simulink model "Resilient-MPC"  (R2018b)
settings: Solver=VariableStepAuto  StartTime=0.0  StopTime=10  RelTol=1e-3
values from neighbouring files (symbols this model uses):
  F = [F,S]    [Initialization.m]
  O = [O;(C*A^(i-1))]    [Initialization.m]
  p = kron(L,pp)    [Initialization.m]
undefined symbols (not defined in the file or in its folder): sigbuilder_block
settings Model: Creator=lenovo  LastModifiedBy=lenovo

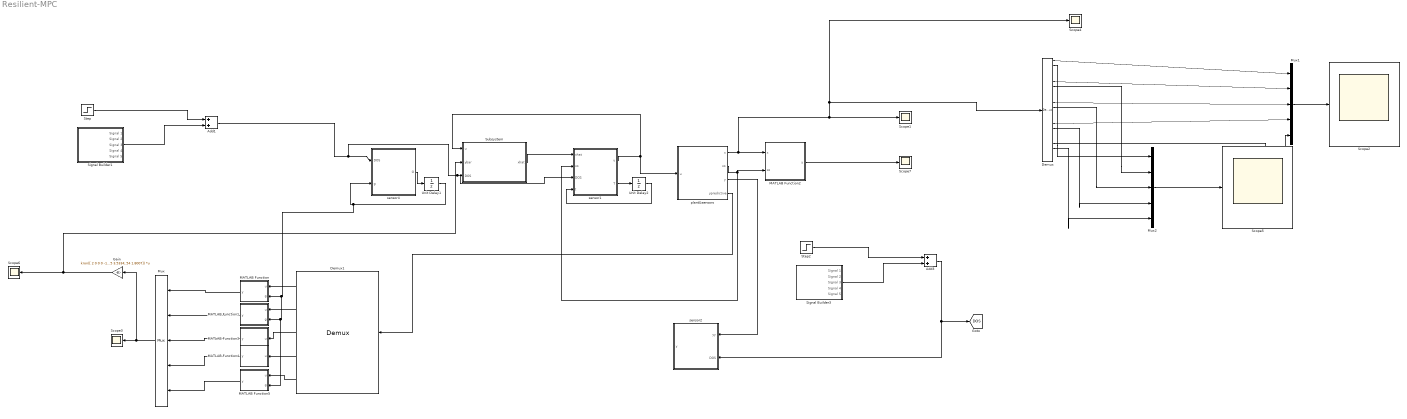
== system Resilient-MPC ==
  Add1 : Sum
  Add3 : Sum
  Demux : Demux  Outputs=20
  Demux1 : Demux  Outputs=5
  Gain : Gain  Gain=kron([ 2 0 0 0 -1; -1 2 0 0 0; -1 0 1 0 0; 0 -1 0 1 0; 0 -1 -1 -1 3],[3.0849 0.6931;2.4258 34.9384;7.0235 3.5334;.54 1.8007])  Multiplication=Matrix(K*u)
  MATLAB Function : MATLAB Function  TreatAsAtomicUnit=on
  MATLAB Function1 : MATLAB Function  TreatAsAtomicUnit=on
  MATLAB Function2 : MATLAB Function  TreatAsAtomicUnit=on
  MATLAB Function3 : MATLAB Function  TreatAsAtomicUnit=on
  MATLAB Function4 : MATLAB Function  TreatAsAtomicUnit=on
  MATLAB Function5 : MATLAB Function  TreatAsAtomicUnit=on
  Mux : Mux  Inputs=5
  Mux1 : Mux  Inputs=5
  Mux2 : Mux  Inputs=5
  Scope{1..7} (7 alike) : Scope
  Signal Builder1 : Subsystem  Tag=STV Subsys  LoadFcn=sigbuilder_block('load');  StartFcn=sigbuilder_block('start');  StopFcn=sigbuilder_block('stop');  ClipboardFcn=sigbuilder_block('clipboard');  mask(Sigbuilder block){tuvar=[0:10]}
      mask help: Simulink:masks:SigbuilderBlock_MD
      mask init:
      | if ~strcmp(get_param(bdroot(gcbh),'SimulationStatus'),'stopped') tuvar = sigbuilder_block('maskInit'); end
      settings: CopyFcn=sigbuilder_block('copy');  DeleteFcn=sigbuilder_block('delete');  ModelCloseFcn=sigbuilder_block('modelClose');  PreSaveFcn=sigbuilder_block('preSave');  PauseFcn=sigbuilder_block('pause');  ContinueFcn=sigbuilder_block('continue');  NameChangeFcn=sigbuilder_block('namechange');  OpenFcn=sigbuilder_block('open',[5.4 30 1141.2 522.6 ]);  CloseFcn=sigbuilder_block('close');
      mask Display: plot(0, 0, 100, 100,[2, 2, 32, 32, 2], [68, 8, 8, 68, 68],[32, 2], [38, 38], [32, 19, 2],[53, 60, 44], [32, 17, 17, 2],[16, 16, 31, 31]);txt = getActiveGroup(gcbh);text(2, 100, txt,'verticalAlignment', 'top');
  Signal Builder3 : Subsystem  Tag=STV Subsys  LoadFcn=sigbuilder_block('load');  StartFcn=sigbuilder_block('start');  StopFcn=sigbuilder_block('stop');  ClipboardFcn=sigbuilder_block('clipboard');  mask(Sigbuilder block){tuvar=[0:10]}
      mask help: Simulink:masks:SigbuilderBlock_MD
      mask init:
      | if ~strcmp(get_param(bdroot(gcbh),'SimulationStatus'),'stopped') tuvar = sigbuilder_block('maskInit'); end
      settings: CopyFcn=sigbuilder_block('copy');  DeleteFcn=sigbuilder_block('delete');  ModelCloseFcn=sigbuilder_block('modelClose');  PreSaveFcn=sigbuilder_block('preSave');  PauseFcn=sigbuilder_block('pause');  ContinueFcn=sigbuilder_block('continue');  NameChangeFcn=sigbuilder_block('namechange');  OpenFcn=sigbuilder_block('open',[5.4 30 1141.2 522.6 ]);  CloseFcn=sigbuilder_block('close');
      mask Display: plot(0, 0, 100, 100,[2, 2, 32, 32, 2], [68, 8, 8, 68, 68],[32, 2], [38, 38], [32, 19, 2],[53, 60, 44], [32, 17, 17, 2],[16, 16, 31, 31]);txt = getActiveGroup(gcbh);text(2, 100, txt,'verticalAlignment', 'top');
  Step : Step  After=-1  SampleTime=10
  Step2 : Step  After=-1  SampleTime=10
  Subsystem : Subsystem
  Unit Delay1 : UnitDelay  InitialCondition=[eye(2) zeros(2,6)]  SampleTime=0.01
  Unit Delay2 : UnitDelay  InitialCondition=[1 0 0 0]  SampleTime=0.01
  plant&sensors : Subsystem
  sensor1 : MATLAB Function  TreatAsAtomicUnit=on
  sensor2 : MATLAB Function  TreatAsAtomicUnit=on
  sensor4 : MATLAB Function  TreatAsAtomicUnit=on
  tag scope: DOS=global
  wires:
  MATLAB Function2/1(y) -> Scope7/1
  sensor1/1(u) -> plant&sensors/1(u), Subsystem/1(u)
  Subsystem/1(xhat) -> sensor1/1(xhat)
  plant&sensors/3(y) -> sensor2/1(yy)
  plant&sensors/2(xo) -> MATLAB Function2/2(xo), sensor1/2(xo)
  Add1/1 -> sensor1/3(DOS), Subsystem/3(DOS), sensor4/1(DOS)
  plant&sensors/4(ypredictive) -> Demux1/1
  sensor4/1(G) -> Unit Delay1/1
  Unit Delay1/1 -> MATLAB Function5/2(g), MATLAB Function1/2(g), MATLAB Function/2(g), sensor4/2(g)
  plant&sensors/1(x) -> Demux/1, Scope4/1, Scope1/1, MATLAB Function2/1(x)
  sensor1/2(T) -> Unit Delay2/1
  Unit Delay2/1 -> sensor1/4(t)
  Step2/1 -> Add3/1
  Signal Builder3/3(Signal 3) -> Add3/2
  Add3/1 -> [DOS], sensor2/2(DOS)
  Step/1 -> Add1/1
  Signal Builder1/3(Signal 3) -> Add1/2
  Demux1/1 -> MATLAB Function/1(u)
  Demux1/2 -> MATLAB Function1/1(u)
  Demux1/3 -> MATLAB Function3/1(u)
  Demux1/4 -> MATLAB Function4/1(u)
  Demux1/5 -> MATLAB Function5/1(u)
  MATLAB Function/1(y) -> Mux/1
  MATLAB Function1/1(y) -> Mux/2
  MATLAB Function3/1(y) -> Mux/3
  MATLAB Function4/1(y) -> Mux/4
  MATLAB Function5/1(y) -> Mux/5
  Mux/1 -> Gain/1, Scope3/1
  Gain/1 -> Subsystem/2(ybar), Scope6/1
  Demux/5 -> Mux1/2
  Demux/17 -> Mux1/5
  Mux1/1 -> Scope2/1
  Demux/13 -> Mux1/4
  Demux/1 -> Mux1/1
  Demux/14 -> Mux2/4
  Demux/9 -> Mux1/3
  Demux/6 -> Mux2/2
  Demux/2 -> Mux2/1
  Demux/10 -> Mux2/3
  Mux2/1 -> Scope5/1
  Demux/18 -> Mux2/5

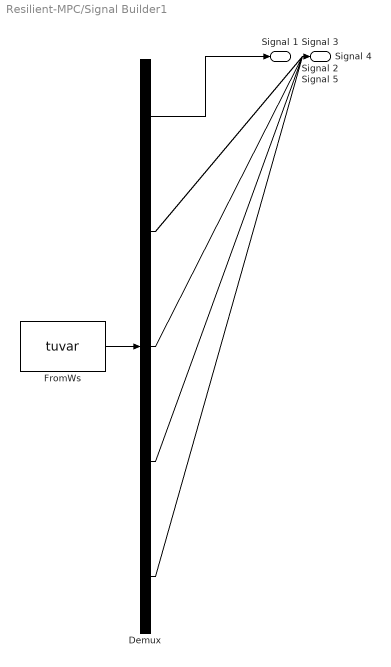
== system Resilient-MPC/Signal Builder1 ==
  Demux : Demux  Tag=STV Demux  Outputs=5
  FromWs : FromWorkspace  Tag=STV FromWs  VariableName=tuvar  SampleTime=0
      SigBuilderData=|
      | common.afterFinalStr = 'Extrapolate'
      | common.sampleTime = 0
      | dataSet.timeRange = [0 10]
      | dataSet.name = 'Group 1'
      | sbobj.Groups.Name = 'Group 1'
      | sbobj.Groups.Signals(1).Name = 'Signal 1'
      | sbobj.Groups.Signals(1).XData = [0 4 4 6 6 10]
      | sbobj.Groups.Signals(1).YData = [0 0 1 1 0 0]
      | sbobj.Groups.Signals(2).Name = 'Signal 2'
      | sbobj.Groups.Signals(2).XData = [0 0.125 0.125 0.25 0.25 0.375 0.375 0.5 0.5 0.625 0.625 0.75 0.75 0.875 0.875 1 1 1.125 1.125 1.25 1.25 1.375 1.375 1.5 1.5 1.625 1.625 1.75 1.75 1.875 1.875 2 2 2.125 2.125 2.25 2.25 2.375 2.375 2.5 2.5 2.625 2.625 2.75 2.75 2.875 2.875 3 3 3.125 3.125 3.25 3.25 3.375 3.375 3.5 3.5 3.625 3.625 3.75 3.75 3.875 3.875 4 4 4.125 4.125 4.25 4.25 4.375 4.375 4.5 4.5 4.625 4.625 4.75 4.75 4.875 4.875 5 5 5.125 5.125 5.25 5.25 5.375 5.375 5.5 5.5 5.625 5.625 5.75 5.75 5.875 5.875 6 6 6.125 6.125 6.25 6.25 6.375 6.375 6.5 6.5 6.625 6.625 6.75 6.75 6.875 6.875 7 7 7.125 7.125 7.25 7.25 7.375 7.375 7.5 7.5 7.625 7.625 7.75 7.75 7.875 7.875 8 8 8.125 8.125 8.25 8.25 8.375 8.375 8.5 8.5 8.625 8.625 8.75 8.75 8.875 8.875 9 9 9.125 9.125 9.25 9.25 9.375 9.375 9.5 9.5 9.625 9.625 9.75 9.75 9.875 9.875 10]
      | sbobj.Groups.Signals(2).YData = [1 1 -1 -1 1 1 -1 -1 1 1 -1 -1 1 1 -1 -1 1 1 -1 -1 1 1 -1 -1 1 1 -1 -1 1 1 -1 -1 1 1 -1 -1 1 1 -1 -1 1 1 -1 -1 1 1 -1 -1 1 1 -1 -1 1 1 -1 -1 1 1 -1 -1 1 1 -1 -1 1 1 -1 -1 1 1 -1 -1 1 1 -1 -1 1 1 -1 -1 1 1 -1 -1 1 1 -1 -1 1 1 -1 -1 1 1 -1 -1 1 1 -1 -1 1 1 -1 -1 1 1 -1 -1 1 1 -1 -1 1 1 -1 -1 1 1 -1 -1 1 1 -1 -1 1 1 -1 -1 1 1 -1 -1 1 1 -1 -1 1 1 -1 -1 1 1 -1 -1 1 1 -1 -1 1 1 -1 -1 1 1 -1 -1 1 1 -1 -1]
      | sbobj.Groups.Signals(3).Name = 'Signal 3'
      | sbobj.Groups.Signals(3).XData = [0 0.16 0.333333333333 0.4 0.4 0.46 0.46 0.833333333333 1 1.005 1.005 1.3 1.3 1.8 1.8 1.9 1.9 2.4 2.4 2.55 2.55 2.625 2.785 2.83333333333 3 3.2 3.2 3.4 3.4 3.5 3.66666666667 3.83333333333 4 4 4.17 4.17 4.33333333333 4.5 4.8 4.8 4.85 4.85 5 5.16666666667 5.33333333333 5.33333333333 5.5 5.5 5.66666666667 5.83333333333 5.83333333333 6 6 6.16666666667 6.33333333333 6.5 6.5 6.66666666667 6.66666666667 6.83333333333 7 7 7.16666666667 7.16666666667 7.33333333333 7.5 7.66666666667 7.83333333333 7.83333333333 8 8 8.16666666667 8.33333333333 8.5 8.5 8.66666666667 8.66666666667 8.83333333333 9 9.16666666667 9.33333333333 9.33333333333 9.5 9.5 9.66666666667 9.83333333333 10]
      | sbobj.Groups.Signals(3).YData = [1 1 1 1 0 0 1 1 1 1 0 0 1 1 0 0 1 1 0 0 1 1 1 1 1 1 0 0 1 1 1 1 1 0 0 1 1 1 1 0 0 1 1 1 1 0 0 1 1 1 0 0 1 1 1 1 0 0 1 1 1 0.005 0.005 1 1 1 1 1 0 0 1 1 1 1 0 0 1 1 1 1 1 0 0 1 1 1 1]
      | sbobj.Groups.Signals(4).Name = 'Signal 4'
      | sbobj.Groups.Signals(4).XData = [0 5 5 10]
      | sbobj.Groups.Signals(4).YData = [0 0 1 1]
      | sbobj.Groups.Signals(5).Name = 'Signal 5'
      | sbobj.Groups.Signals(5).XData = [0 0.45 0.45 0.5 0.5 0.95 0.95 1 1 1.45 1.45 1.5 1.5 1.95 1.95 2 2 2.45 2.45 2.5 2.5 2.95 2.95 3 3 3.45 3.45 3.5 3.5 3.95 3.95 4 4 4.45 4.45 4.5 4.5 4.95 4.95 5 5 5.45 5.45 5.5 5.5 5.95 5.95 6 6 6.45 6.45 6.5 6.5 6.95 6.95 7 7 7.45 7.45 7.5 7.5 7.95 7.95 8 8 8.45 8.45 8.5 8.5 8.95 8.95 9 9 9.45 9.45 9.5 9.5 9.95 9.95 10]
      | sbobj.Groups.Signals(5).YData = [1 1 0 0 1 1 0 0 1 1 0 0 1 1 0 0 1 1 0 0 1 1 0 0 1 1 0 0 1 1 0 0 1 1 0 0 1 1 0 0 1 1 0 0 1 1 0 0 1 1 0 0 1 1 0 0 1 1 0 0 1 1 0 0 1 1 0 0 1 1 0 0 1 1 0 0 0.995 0.995 0 0]
  Signal 1 : Outport  Tag=STV Outport
  Signal 2 : Outport  Tag=STV Outport  Port=2
  Signal 3 : Outport  Tag=STV Outport  Port=3
  Signal 4 : Outport  Tag=STV Outport  Port=4
  Signal 5 : Outport  Tag=STV Outport  Port=5
  wires:
  Demux/1 -> Signal 1/1
  FromWs/1 -> Demux/1
  Demux/2 -> Signal 2/1
  Demux/3 -> Signal 3/1
  Demux/4 -> Signal 4/1
  Demux/5 -> Signal 5/1

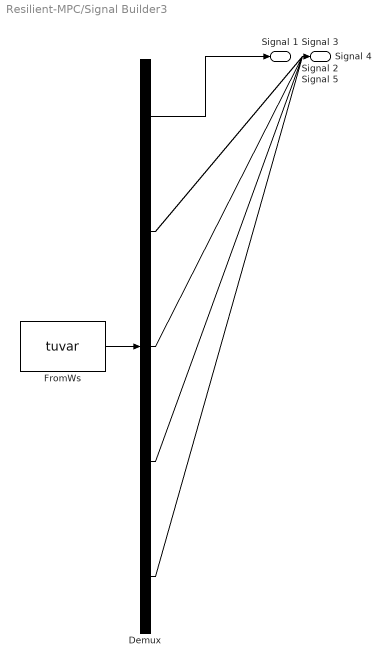
== system Resilient-MPC/Signal Builder3 ==
  Demux : Demux  Tag=STV Demux  Outputs=5
  FromWs : FromWorkspace  Tag=STV FromWs  VariableName=tuvar  SampleTime=0
      SigBuilderData=|
      | common.afterFinalStr = 'Extrapolate'
      | common.sampleTime = 0
      | dataSet.timeRange = [0 10]
      | dataSet.name = 'Group 1'
      | sbobj.Groups.Name = 'Group 1'
      | sbobj.Groups.Signals(1).Name = 'Signal 1'
      | sbobj.Groups.Signals(1).XData = [0 4 4 6 6 10]
      | sbobj.Groups.Signals(1).YData = [0 0 1 1 0 0]
      | sbobj.Groups.Signals(2).Name = 'Signal 2'
      | sbobj.Groups.Signals(2).XData = [0 0.125 0.125 0.25 0.25 0.375 0.375 0.5 0.5 0.625 0.625 0.75 0.75 0.875 0.875 1 1 1.125 1.125 1.25 1.25 1.375 1.375 1.5 1.5 1.625 1.625 1.75 1.75 1.875 1.875 2 2 2.125 2.125 2.25 2.25 2.375 2.375 2.5 2.5 2.625 2.625 2.75 2.75 2.875 2.875 3 3 3.125 3.125 3.25 3.25 3.375 3.375 3.5 3.5 3.625 3.625 3.75 3.75 3.875 3.875 4 4 4.125 4.125 4.25 4.25 4.375 4.375 4.5 4.5 4.625 4.625 4.75 4.75 4.875 4.875 5 5 5.125 5.125 5.25 5.25 5.375 5.375 5.5 5.5 5.625 5.625 5.75 5.75 5.875 5.875 6 6 6.125 6.125 6.25 6.25 6.375 6.375 6.5 6.5 6.625 6.625 6.75 6.75 6.875 6.875 7 7 7.125 7.125 7.25 7.25 7.375 7.375 7.5 7.5 7.625 7.625 7.75 7.75 7.875 7.875 8 8 8.125 8.125 8.25 8.25 8.375 8.375 8.5 8.5 8.625 8.625 8.75 8.75 8.875 8.875 9 9 9.125 9.125 9.25 9.25 9.375 9.375 9.5 9.5 9.625 9.625 9.75 9.75 9.875 9.875 10]
      | sbobj.Groups.Signals(2).YData = [1 1 -1 -1 1 1 -1 -1 1 1 -1 -1 1 1 -1 -1 1 1 -1 -1 1 1 -1 -1 1 1 -1 -1 1 1 -1 -1 1 1 -1 -1 1 1 -1 -1 1 1 -1 -1 1 1 -1 -1 1 1 -1 -1 1 1 -1 -1 1 1 -1 -1 1 1 -1 -1 1 1 -1 -1 1 1 -1 -1 1 1 -1 -1 1 1 -1 -1 1 1 -1 -1 1 1 -1 -1 1 1 -1 -1 1 1 -1 -1 1 1 -1 -1 1 1 -1 -1 1 1 -1 -1 1 1 -1 -1 1 1 -1 -1 1 1 -1 -1 1 1 -1 -1 1 1 -1 -1 1 1 -1 -1 1 1 -1 -1 1 1 -1 -1 1 1 -1 -1 1 1 -1 -1 1 1 -1 -1 1 1 -1 -1 1 1 -1 -1]
      | sbobj.Groups.Signals(3).Name = 'Signal 3'
      | sbobj.Groups.Signals(3).XData = [0 0.16 0.333333333333 0.4 0.4 0.46 0.46 0.833333333333 1 1.005 1.005 1.3 1.3 1.8 1.8 1.9 1.9 2.4 2.4 2.55 2.55 2.625 2.785 2.83333333333 3 3.2 3.2 3.4 3.4 3.5 3.66666666667 3.83333333333 4 4 4.17 4.17 4.33333333333 4.5 4.8 4.8 4.85 4.85 5 5.16666666667 5.33333333333 5.33333333333 5.5 5.5 5.66666666667 5.83333333333 5.83333333333 6 6 6.16666666667 6.33333333333 6.5 6.5 6.66666666667 6.66666666667 6.83333333333 7 7 7.16666666667 7.16666666667 7.33333333333 7.5 7.66666666667 7.83333333333 7.83333333333 8 8 8.16666666667 8.33333333333 8.5 8.5 8.66666666667 8.66666666667 8.83333333333 9 9.16666666667 9.33333333333 9.33333333333 9.5 9.5 9.66666666667 9.83333333333 10]
      | sbobj.Groups.Signals(3).YData = [1 1 1 1 0 0 1 1 1 1 0 0 1 1 0 0 1 1 0 0 1 1 1 1 1 1 0 0 1 1 1 1 1 0 0 1 1 1 1 0 0 1 1 1 1 0 0 1 1 1 0 0 1 1 1 1 0 0 1 1 1 0.005 0.005 1 1 1 1 1 0 0 1 1 1 1 0 0 1 1 1 1 1 0 0 1 1 1 1]
      | sbobj.Groups.Signals(4).Name = 'Signal 4'
      | sbobj.Groups.Signals(4).XData = [0 5 5 10]
      | sbobj.Groups.Signals(4).YData = [0 0 1 1]
      | sbobj.Groups.Signals(5).Name = 'Signal 5'
      | sbobj.Groups.Signals(5).XData = [0 0.45 0.45 0.5 0.5 0.95 0.95 1 1 1.45 1.45 1.5 1.5 1.95 1.95 2 2 2.45 2.45 2.5 2.5 2.95 2.95 3 3 3.45 3.45 3.5 3.5 3.95 3.95 4 4 4.45 4.45 4.5 4.5 4.95 4.95 5 5 5.45 5.45 5.5 5.5 5.95 5.95 6 6 6.45 6.45 6.5 6.5 6.95 6.95 7 7 7.45 7.45 7.5 7.5 7.95 7.95 8 8 8.45 8.45 8.5 8.5 8.95 8.95 9 9 9.45 9.45 9.5 9.5 9.95 9.95 10]
      | sbobj.Groups.Signals(5).YData = [1 1 0 0 1 1 0 0 1 1 0 0 1 1 0 0 1 1 0 0 1 1 0 0 1 1 0 0 1 1 0 0 1 1 0 0 1 1 0 0 1 1 0 0 1 1 0 0 1 1 0 0 1 1 0 0 1 1 0 0 1 1 0 0 1 1 0 0 1 1 0 0 1 1 0 0 0.995 0.995 0 0]
  Signal 1 : Outport  Tag=STV Outport
  Signal 2 : Outport  Tag=STV Outport  Port=2
  Signal 3 : Outport  Tag=STV Outport  Port=3
  Signal 4 : Outport  Tag=STV Outport  Port=4
  Signal 5 : Outport  Tag=STV Outport  Port=5
  wires:
  Demux/1 -> Signal 1/1
  FromWs/1 -> Demux/1
  Demux/2 -> Signal 2/1
  Demux/3 -> Signal 3/1
  Demux/4 -> Signal 4/1
  Demux/5 -> Signal 5/1

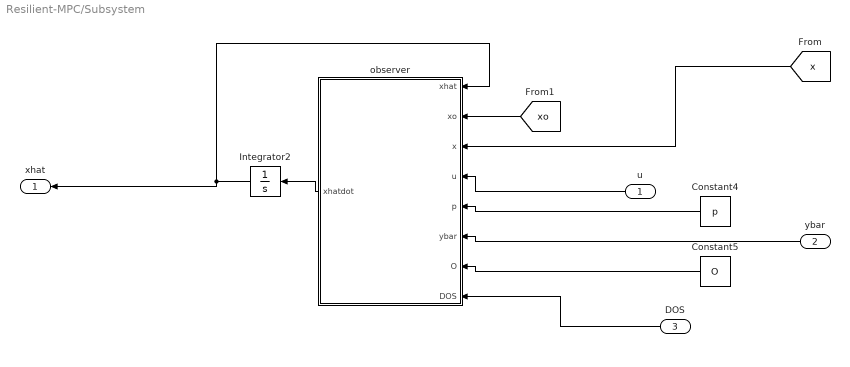
== system Resilient-MPC/Subsystem ==
  u : Inport
  ybar : Inport  Port=2
  DOS : Inport  Port=3
  Constant4 : Constant  Value=p
  Constant5 : Constant  Value=O
  Integrator2 : Integrator  InitialCondition=[-10;-9;-8;-7;-6;5;-4;-3;-2;-1;1;2;3;4;5;6;7;8;9;10]
  observer : MATLAB Function  TreatAsAtomicUnit=on
  xhat : Outport
  wires:
  observer/1(xhatdot) -> Integrator2/1
  Constant4/1 -> observer/5(p)
  Integrator2/1 -> observer/1(xhat), xhat/1
  Constant5/1 -> observer/7(O)
  u/1 -> observer/4(u)
  ybar/1 -> observer/6(ybar)
  DOS/1 -> observer/8(DOS)
  [xo] -> observer/2(xo)
  [x] -> observer/3(x)

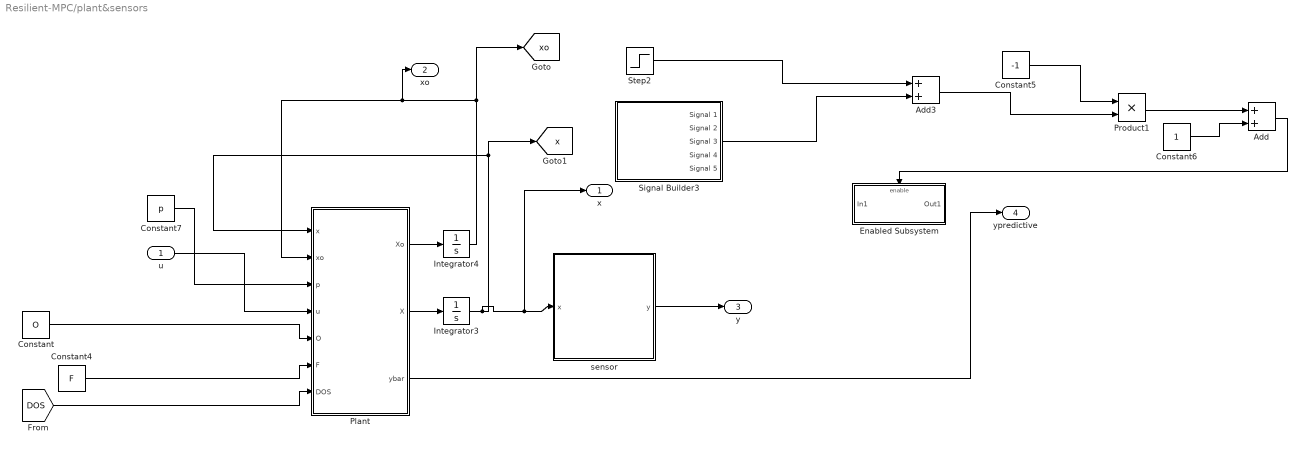
== system Resilient-MPC/plant&sensors ==
  u : Inport
  Add : Sum
  Add3 : Sum
  Constant : Constant  Value=O
  Constant4 : Constant  Value=F
  Constant5 : Constant  Value=-1
  Constant6 : Constant
  Constant7 : Constant  Value=p
  Enabled Subsystem : Subsystem  TreatAsAtomicUnit=on
  Integrator3 : Integrator  InitialCondition=[-10;-9;-8;-7;-6;5;-4;-3;-2;-1;1;2;3;4;5;6;7;8;9;10]
  Integrator4 : Integrator  InitialCondition=[-5;1;3;-15]
  Plant : MATLAB Function  TreatAsAtomicUnit=on
  Product1 : Product
  Signal Builder3 : Subsystem  Tag=STV Subsys  LoadFcn=sigbuilder_block('load');  StartFcn=sigbuilder_block('start');  StopFcn=sigbuilder_block('stop');  ClipboardFcn=sigbuilder_block('clipboard');  mask(Sigbuilder block){tuvar=[0:10]}
      mask help: Simulink:masks:SigbuilderBlock_MD
      mask init:
      | if ~strcmp(get_param(bdroot(gcbh),'SimulationStatus'),'stopped') tuvar = sigbuilder_block('maskInit'); end
      settings: CopyFcn=sigbuilder_block('copy');  DeleteFcn=sigbuilder_block('delete');  ModelCloseFcn=sigbuilder_block('modelClose');  PreSaveFcn=sigbuilder_block('preSave');  PauseFcn=sigbuilder_block('pause');  ContinueFcn=sigbuilder_block('continue');  NameChangeFcn=sigbuilder_block('namechange');  OpenFcn=sigbuilder_block('open',[5.4 30 1141.2 522.6 ]);  CloseFcn=sigbuilder_block('close');
      mask Display: plot(0, 0, 100, 100,[2, 2, 32, 32, 2], [68, 8, 8, 68, 68],[32, 2], [38, 38], [32, 19, 2],[53, 60, 44], [32, 17, 17, 2],[16, 16, 31, 31]);txt = getActiveGroup(gcbh);text(2, 100, txt,'verticalAlignment', 'top');
  Step2 : Step  After=-1  SampleTime=10
  sensor : MATLAB Function  TreatAsAtomicUnit=on
  x : Outport
  xo : Outport  Port=2
  y : Outport  Port=3
  ypredictive : Outport  Port=4
  tag scope: x=global, xo=global
  wires:
  sensor/1(y) -> y/1
  Plant/1(Xo) -> Integrator4/1
  Plant/2(X) -> Integrator3/1
  Constant/1 -> Plant/5(O)
  Integrator4/1 -> [xo], xo/1, Plant/2(xo)
  Integrator3/1 -> [x], Plant/1(x), x/1, sensor/1(x)
  u/1 -> Plant/4(u)
  Constant4/1 -> Plant/6(F)
  Step2/1 -> Add3/1
  Signal Builder3/3(Signal 3) -> Add3/2
  Constant6/1 -> Add/2
  Product1/1 -> Add/1
  Constant5/1 -> Product1/1
  Add3/1 -> Product1/2
  Add/1 -> Enabled Subsystem/Enable
  Constant7/1 -> Plant/3(p)
  Plant/3(ybar) -> ypredictive/1
  [DOS] -> Plant/7(DOS)

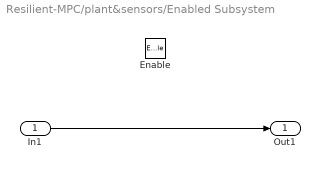
== system Resilient-MPC/plant&sensors/Enabled Subsystem ==
  In1 : Inport
  Enable : EnablePort
  Out1 : Outport
  wires:
  In1/1 -> Out1/1

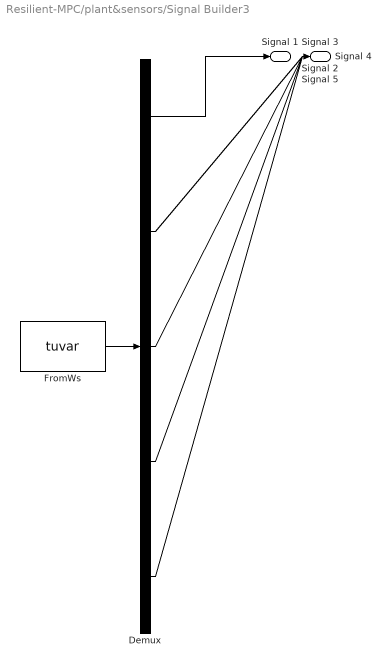
== system Resilient-MPC/plant&sensors/Signal Builder3 ==
  Demux : Demux  Tag=STV Demux  Outputs=5
  FromWs : FromWorkspace  Tag=STV FromWs  VariableName=tuvar  SampleTime=0
      SigBuilderData=|
      | common.afterFinalStr = 'Extrapolate'
      | common.sampleTime = 0
      | dataSet.timeRange = [0 10]
      | dataSet.name = 'Group 1'
      | sbobj.Groups.Name = 'Group 1'
      | sbobj.Groups.Signals(1).Name = 'Signal 1'
      | sbobj.Groups.Signals(1).XData = [0 4 4 6 6 10]
      | sbobj.Groups.Signals(1).YData = [0 0 1 1 0 0]
      | sbobj.Groups.Signals(2).Name = 'Signal 2'
      | sbobj.Groups.Signals(2).XData = [0 0.125 0.125 0.25 0.25 0.375 0.375 0.5 0.5 0.625 0.625 0.75 0.75 0.875 0.875 1 1 1.125 1.125 1.25 1.25 1.375 1.375 1.5 1.5 1.625 1.625 1.75 1.75 1.875 1.875 2 2 2.125 2.125 2.25 2.25 2.375 2.375 2.5 2.5 2.625 2.625 2.75 2.75 2.875 2.875 3 3 3.125 3.125 3.25 3.25 3.375 3.375 3.5 3.5 3.625 3.625 3.75 3.75 3.875 3.875 4 4 4.125 4.125 4.25 4.25 4.375 4.375 4.5 4.5 4.625 4.625 4.75 4.75 4.875 4.875 5 5 5.125 5.125 5.25 5.25 5.375 5.375 5.5 5.5 5.625 5.625 5.75 5.75 5.875 5.875 6 6 6.125 6.125 6.25 6.25 6.375 6.375 6.5 6.5 6.625 6.625 6.75 6.75 6.875 6.875 7 7 7.125 7.125 7.25 7.25 7.375 7.375 7.5 7.5 7.625 7.625 7.75 7.75 7.875 7.875 8 8 8.125 8.125 8.25 8.25 8.375 8.375 8.5 8.5 8.625 8.625 8.75 8.75 8.875 8.875 9 9 9.125 9.125 9.25 9.25 9.375 9.375 9.5 9.5 9.625 9.625 9.75 9.75 9.875 9.875 10]
      | sbobj.Groups.Signals(2).YData = [1 1 -1 -1 1 1 -1 -1 1 1 -1 -1 1 1 -1 -1 1 1 -1 -1 1 1 -1 -1 1 1 -1 -1 1 1 -1 -1 1 1 -1 -1 1 1 -1 -1 1 1 -1 -1 1 1 -1 -1 1 1 -1 -1 1 1 -1 -1 1 1 -1 -1 1 1 -1 -1 1 1 -1 -1 1 1 -1 -1 1 1 -1 -1 1 1 -1 -1 1 1 -1 -1 1 1 -1 -1 1 1 -1 -1 1 1 -1 -1 1 1 -1 -1 1 1 -1 -1 1 1 -1 -1 1 1 -1 -1 1 1 -1 -1 1 1 -1 -1 1 1 -1 -1 1 1 -1 -1 1 1 -1 -1 1 1 -1 -1 1 1 -1 -1 1 1 -1 -1 1 1 -1 -1 1 1 -1 -1 1 1 -1 -1 1 1 -1 -1]
      | sbobj.Groups.Signals(3).Name = 'Signal 3'
      | sbobj.Groups.Signals(3).XData = [0 0.16 0.333333333333 0.4 0.4 0.46 0.46 0.833333333333 1 1.005 1.005 1.3 1.3 1.8 1.8 1.9 1.9 2.4 2.4 2.55 2.55 2.625 2.785 2.83333333333 3 3.2 3.2 3.4 3.4 3.5 3.66666666667 3.83333333333 4 4 4.17 4.17 4.33333333333 4.5 4.8 4.8 4.85 4.85 5 5.16666666667 5.33333333333 5.33333333333 5.5 5.5 5.66666666667 5.83333333333 5.83333333333 6 6 6.16666666667 6.33333333333 6.5 6.5 6.66666666667 6.66666666667 6.83333333333 7 7 7.16666666667 7.16666666667 7.33333333333 7.5 7.66666666667 7.83333333333 7.83333333333 8 8 8.16666666667 8.33333333333 8.5 8.5 8.66666666667 8.66666666667 8.83333333333 9 9.16666666667 9.33333333333 9.33333333333 9.5 9.5 9.66666666667 9.83333333333 10]
      | sbobj.Groups.Signals(3).YData = [1 1 1 1 0 0 1 1 1 1 0 0 1 1 0 0 1 1 0 0 1 1 1 1 1 1 0 0 1 1 1 1 1 0 0 1 1 1 1 0 0 1 1 1 1 0 0 1 1 1 0 0 1 1 1 1 0 0 1 1 1 0.005 0.005 1 1 1 1 1 0 0 1 1 1 1 0 0 1 1 1 1 1 0 0 1 1 1 1]
      | sbobj.Groups.Signals(4).Name = 'Signal 4'
      | sbobj.Groups.Signals(4).XData = [0 5 5 10]
      | sbobj.Groups.Signals(4).YData = [0 0 1 1]
      | sbobj.Groups.Signals(5).Name = 'Signal 5'
      | sbobj.Groups.Signals(5).XData = [0 0.45 0.45 0.5 0.5 0.95 0.95 1 1 1.45 1.45 1.5 1.5 1.95 1.95 2 2 2.45 2.45 2.5 2.5 2.95 2.95 3 3 3.45 3.45 3.5 3.5 3.95 3.95 4 4 4.45 4.45 4.5 4.5 4.95 4.95 5 5 5.45 5.45 5.5 5.5 5.95 5.95 6 6 6.45 6.45 6.5 6.5 6.95 6.95 7 7 7.45 7.45 7.5 7.5 7.95 7.95 8 8 8.45 8.45 8.5 8.5 8.95 8.95 9 9 9.45 9.45 9.5 9.5 9.95 9.95 10]
      | sbobj.Groups.Signals(5).YData = [1 1 0 0 1 1 0 0 1 1 0 0 1 1 0 0 1 1 0 0 1 1 0 0 1 1 0 0 1 1 0 0 1 1 0 0 1 1 0 0 1 1 0 0 1 1 0 0 1 1 0 0 1 1 0 0 1 1 0 0 1 1 0 0 1 1 0 0 1 1 0 0 1 1 0 0 0.995 0.995 0 0]
  Signal 1 : Outport  Tag=STV Outport
  Signal 2 : Outport  Tag=STV Outport  Port=2
  Signal 3 : Outport  Tag=STV Outport  Port=3
  Signal 4 : Outport  Tag=STV Outport  Port=4
  Signal 5 : Outport  Tag=STV Outport  Port=5
  wires:
  Demux/1 -> Signal 1/1
  FromWs/1 -> Demux/1
  Demux/2 -> Signal 2/1
  Demux/3 -> Signal 3/1
  Demux/4 -> Signal 4/1
  Demux/5 -> Signal 5/1

== matlab function Resilient-MPC/Subsystem/observer ==
  data: xhat input; xo input; x input; xhatdot output; u input; p input; ybar input; O input; DOS input
function xhatdot = fcn(xhat,xo,x,u,p,ybar,O,DOS)
A=[0 1 0 0;-48.6 -1.26 48.6 0;0 0 0 10; 1.95 0 -1.95 0];
B=[0;21.6;0;0];
C=[1 0 1 -1;0 1 0 0];
teta=5;
H=[3.0849 0.6931;2.4258 34.9384;7.0235 3.5334;.54 1.8007];


%Lo=[0 0 0 0 0 0;-1 2-DOS 0 0 0 -1+DOS;-1+DOS -1 2-DOS 0 0 0;0 -1+DOS 0 1-DOS 0 0;0 0 -1 0 1 0;0 0 -1+DOS -1 -1 3-DOS];
% L=[0 0 0 0 0 0;-1 2 0 0 0 -1;-1 -1 2 0 0 0;0 -1 0 1 0 0;0 0 -1 0 1 0;0 0 -1 -1 -1 3];
L=[ 2 0 0 0 -1; -1 2 0 0 0; -1 0 1 0 0; 0 -1 0 1 0; 0 -1 -1 -1 3];
B_bar=[1.08e-05
       0.02159
 1.755e-11
  7.018e-09];
N=5;
A0=kron(eye(N),A);
z2=kron(L,H*C);
B0=kron(eye(N),B);
Hsigma=[H zeros(4,6)];
Fbar=[B_bar zeros(4,3)];
C0=kron(eye(5),C);

H0=kron(eye(5),H);
Fbar0=kron(eye(5),Fbar);


H=[eye(2) zeros(2,6)];
    H0=kron(eye(5),H);
%   xhatdot=A0*xhat+Fbar0*ubar+teta*(ybar-kron(L,Hsigma*O)*xhat);
if DOS==1
%  xhatdot= A0*xhat+B0*u+teta*(ybar-z2*xhat);
xhatdot= A0*xhat+B0*u+teta*(ybar-z2*xhat);
else
FF=p;
e=kron(ones(5,1),xo)-x;
ubar=FF*e;
xhatdot=A0*xhat+Fbar0*ubar+teta*(ybar-kron(L,Hsigma*O)*xhat);
end

== matlab function Resilient-MPC/MATLAB Function ==
  data: u input; y output; g input
function y = fcn(u,g)

y =g*u;

== matlab function Resilient-MPC/sensor1 ==
  data: xhat input; u output; xo input; DOS input; t input; T output
function [u,T]  = fcn(xhat,xo,DOS,t)
c=2;
Lu=[-1 2 0 0 0 -1;-1 -1 2 0 0 0;0 -1 0 1 0 0;0 0 -1 0 1 0;0 0 -1 -1 -1 3];
A=[0.9976    0.0099    0.0024    0.0001
   -0.4824    0.9851    0.4824    0.0242
    0.0010    0.0000    0.9990    0.1000
    0.0195    0.0001   -0.0195    0.9990];
B=[0.0011
    0.2145
    0.0000
    0.0000];
q=[1.1926    0.4512   -0.9407    1.5229];
p=[];
Np=4;
for i=0:Np-1
    p1=-c*q*(A-B*q)^i;
    p=[p ;p1];
end


if DOS==0
  T=[1 0 0 0];
else
 
  T=circshift(t',1,2)
end
 K=t'*p;
Z=kron(Lu,K);
u=Z*[xo;xhat];

== matlab function Resilient-MPC/plant&sensors/sensor ==
  data: x input; y output
function y  = fcn(x)
C=[1 0 1 -1;0 1 0 0];
N=5;
C0=kron(eye(N),C);
y=C0*x;

== matlab function Resilient-MPC/sensor2 ==
  data: yy input; y output; DOS input
function y = fcn(yy,DOS)
Lo=[ 2-DOS 0 0 0 -1+DOS; -1 2-DOS 0 0 0; -1+DOS 0 1-DOS 0 0; 0 -1 0 1 0; 0 -1+DOS -1 -1 3-DOS];
H=[3.0849 0.6931;2.4258 34.9384;7.0235 3.5334;.54 1.8007];
L=[ 2 0 0 0 -1; -1 2 0 0 0; -1 0 1 0 0; 0 -1 0 1 0; 0 -1 -1 -1 3];
y=kron(Lo,H)*yy;

== matlab function Resilient-MPC/plant&sensors/Plant ==
  data: Xo output; x input; xo input; p input; u input; X output; O input; F input; DOS input; ybar output
function [Xo,X,ybar] = fcn(x,xo,p,u,O,F,DOS)
A=[0 1 0 0;-48.6 -1.26 48.6 0;0 0 0 10; 1.95 0 -1.95 0];
B=[0;21.6;0;0];
A0=kron(eye(5),A);
B0=kron(eye(5),B);
O0=kron(eye(5),O);
F0=kron(eye(5),F);

% ybar = O0*x+sigma0*wbar+dbar+F0*ubar;
if DOS==1
    FF=p;
e=kron(ones(5,1),xo)-x;
ubar=FF*e;
   ybar = O0*x+F0*ubar; 
else
 ybar = O0*x;
end
Xo =A*xo;
X=A0*x+B0*u;

== matlab function Resilient-MPC/MATLAB Function1 ==
  data: u input; y output; g input
function y = fcn(u,g)

y =g*u;

== matlab function Resilient-MPC/MATLAB Function2 ==
  data: x input; y output; xo input
function y = fcn(x,xo)
y=norm(kron(ones(5,1),xo)-x);

== matlab function Resilient-MPC/sensor4 ==
  data: DOS input; g input; G output
function G  = fcn(DOS,g)
Lo=[ 2-DOS 0 0 0 -1+DOS; -1 2-DOS 0 0 0; -1+DOS 0 1-DOS 0 0; 0 -1 0 1 0; 0 -1+DOS -1 -1 3-DOS];
H=[3.0849 0.6931;2.4258 34.9384;7.0235 3.5334;.54 1.8007];
L=[ 2 0 0 0 -1; -1 2 0 0 0; -1 0 1 0 0; 0 -1 0 1 0; 0 -1 -1 -1 3];
if DOS==0
G=[eye(2) zeros(2,6)];

else
   G=circshift(g,2,2);
end
 G0=kron(eye(5),g);

== matlab function Resilient-MPC/MATLAB Function3 ==
  data: u input; y output
function y = fcn(u)

y =[eye(2) zeros(2,6)]*u;

== matlab function Resilient-MPC/MATLAB Function4 ==
  data: u input; y output
function y = fcn(u)

y =[eye(2) zeros(2,6)]*u;

== matlab function Resilient-MPC/MATLAB Function5 ==
  data: u input; y output; g input
function y = fcn(u,g)

y =g*u;
